simulink model "modelo"  (R2025b)
settings: Solver=ode45  StartTime=0.0  StopTime=14  RelTol=1e-3  EnableMultiTasking=on
undefined symbols (not defined in the file): param
settings Model: Creator=Guillermo  LastModifiedBy=franco
settings SolverCC: AlgebraicLoopSolver=TrustRegion
settings DataIOCC: LimitDataPoints=on  SaveFormat=Array  SignalLoggingSaveFormat=ModelDataLogs  ReturnWorkspaceOutputs=off
settings OptimizationCC: ExpressionDepthLimit=2147483647.0  InitFltsAndDblsToZero=on  LifeSpan=inf
settings DebuggingCC: SaveWithParameterizedLinksMsg=none  UnderspecifiedInitializationDetection=Classic  MergeDetectMultiDrivingBlocksExec=none  SignalResolutionControl=TryResolveAllWithWarning  SolverPrmCheckMsg=warning  MultiTaskDSMMsg=warning  MultiTaskCondExecSysMsg=none  FcnCallInpInsideContextMsg=warning  UnconnectedInputMsg=warning  UnconnectedOutputMsg=warning  UnconnectedLineMsg=warning  StateNameClashWarn=warning  SFUnexpectedBacktrackingDiag=warning  SFNoUnconditionalDefaultTransitionDiag=warning  SFExecutionAtInitializationDiag=none  ArithmeticOperatorsInVariantConditions=warning
settings HardwareCC: ProdBitPerPointer=32.0  ProdBitPerSizeT=32.0  ProdBitPerPtrDiffT=32.0  ProdLargestAtomicFloat=None  ProdIntDivRoundTo=Undefined  ProdEndianess=Unspecified  ProdWordSize=32.0  ProdHWDeviceType=32-bit Generic
settings ModelReferenceCC: PropagateSignalLabelsOutOfModel=off
settings SFSimCC: SimUseLocalCustomCode=off  CustomCodeUndefinedFunction=UseInterfaceOnly
settings RTWCC: RTWUseLocalCustomCode=off  GPUComputeCapability=3.5
settings CodeAppCC: StateflowObjectComments=on
settings GRTTargetCC: TargetFcnLib=ansi_tfl_tmw.mat  TargetLangStandard=C89/C90 (ANSI)  CombineOutputUpdateFcns=off  GRTInterface=on
settings ConfigComp: CovMetricSettings=dw  CovSaveCumulativeToWorkspaceVar=on  CovSaveSingleToWorkspaceVar=on  CovExternalEMLEnable=off

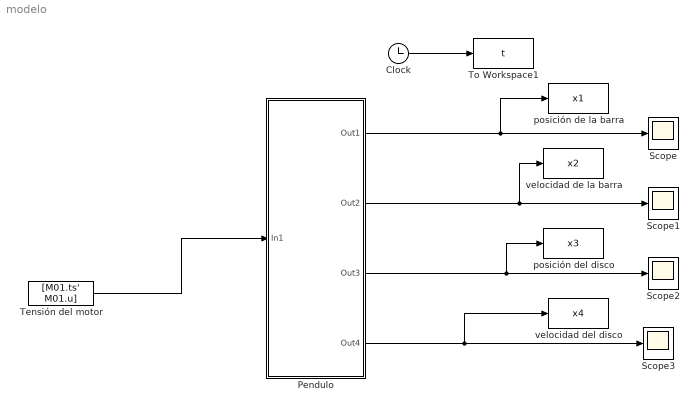
== system modelo ==
  Clock : Clock
  Pendulo : Subsystem
  Scope{,1..3} (4 alike) : Scope
      Scope settings: ActiveDisplayYMinimum=-1.4802014068199523  ActiveDisplayYMaximum=1.3877329973868153
      Scope1 settings: ActiveDisplayYMinimum=-6.9139958886742932  ActiveDisplayYMaximum=7.2975474464828647
      Scope2 settings: ActiveDisplayYMinimum=-17.804918784606386  ActiveDisplayYMaximum=83.795104863164056  DataLoggingVariableName=ScopeData2
      Scope3 settings: ActiveDisplayYMinimum=-110.83164635850608  ActiveDisplayYMaximum=131.3400190514694  DataLoggingVariableName=ScopeData3
  Tensión del motor : FromWorkspace  VariableName=[M01.ts' M01.u]  SampleTime=0.01  ZeroCross=off
  To Workspace1 : ToWorkspace  VariableName=t  SampleTime=-1
  posición de la barra : ToWorkspace  VariableName=x1  SampleTime=-1
  posición del disco : ToWorkspace  VariableName=x3  SampleTime=-1
  velocidad de la barra : ToWorkspace  VariableName=x2  SampleTime=-1
  velocidad del disco : ToWorkspace  VariableName=x4  SampleTime=-1
  wires:
  Clock/1 -> To Workspace1/1
  Tensión del motor/1 -> Pendulo/1(In1)
  Pendulo/1(Out1) -> posición de la barra/1, Scope/1
  Pendulo/2(Out2) -> velocidad de la barra/1, Scope1/1
  Pendulo/3(Out3) -> Scope2/1, posición del disco/1
  Pendulo/4(Out4) -> Scope3/1, velocidad del disco/1

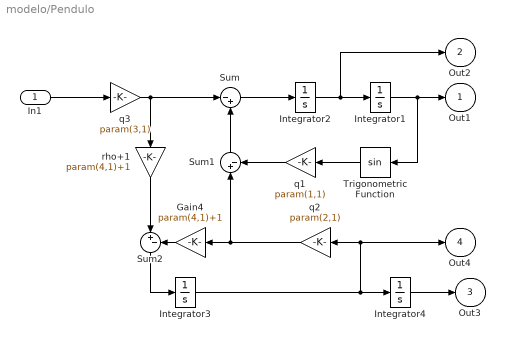
== system modelo/Pendulo ==
  In1 : Inport
  Gain4 : Gain  Gain=param(4,1)+1
  Integrator{1..4} (4 alike) : Integrator
  Sum : Sum  Inputs=|-+
  Sum1 : Sum  Inputs=|+-
  Sum2 : Sum  Inputs=|+-
  Trigonometric Function : Trigonometry
  q1 : Gain  Gain=param(1,1)
  q2 : Gain  Gain=param(2,1)
  q3 : Gain  Gain=param(3,1)
  rho+1 : Gain  Gain=param(4,1)+1
  Out1 : Outport
  Out2 : Outport  Port=2
  Out3 : Outport  Port=3
  Out4 : Outport  Port=4
  wires:
  q1/1 -> Sum1/2
  Trigonometric Function/1 -> q1/1
  Integrator1/1 -> Out1/1, Trigonometric Function/1
  Integrator2/1 -> Out2/1, Integrator1/1
  Sum/1 -> Integrator2/1
  Sum1/1 -> Sum/2
  q3/1 -> rho+1/1, Sum/1
  In1/1 -> q3/1
  q2/1 -> Sum1/1, Gain4/1
  Gain4/1 -> Sum2/2
  rho+1/1 -> Sum2/1
  Sum2/1 -> Integrator3/1
  Integrator3/1 -> Out4/1, q2/1, Integrator4/1
  Integrator4/1 -> Out3/1
